simulink model "lab6"  (Simulink 7.7)
settings: Solver=ode45  StartTime=0.0  StopTime=10.0  RelTol=1e-3
settings Model: Creator=Muhammad Ali khan  LastModifiedBy=Muhammad Ali khan

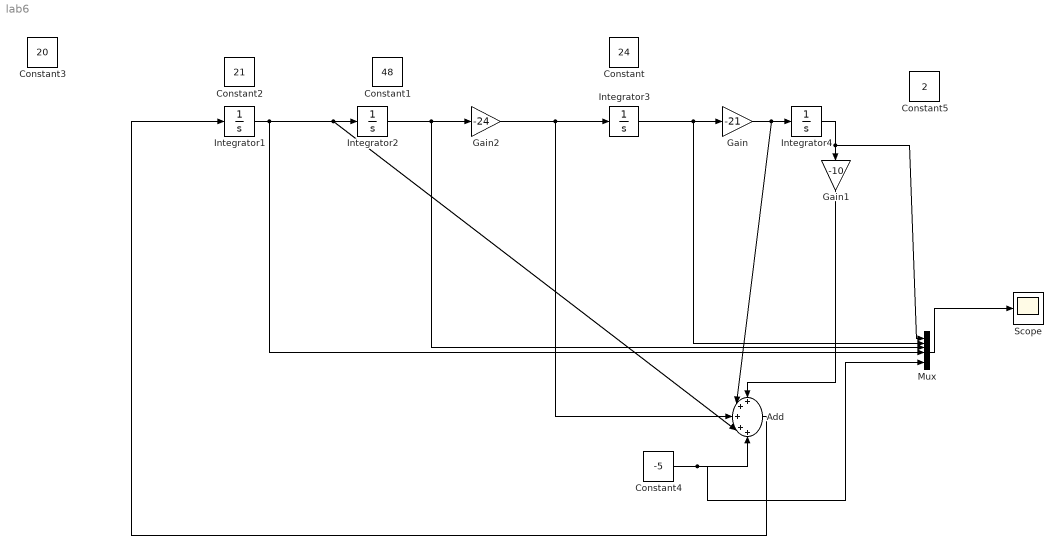
== system lab6 ==
  Add : Sum  Inputs=+++++
  Constant : Constant  Value=24
  Constant1 : Constant  Value=48
  Constant2 : Constant  Value=21
  Constant3 : Constant  Value=20
  Constant4 : Constant  Value=-5
  Constant5 : Constant  Value=2
  Gain : Gain  Gain=-21
  Gain1 : Gain  Gain=-10
  Gain2 : Gain  Gain=-24
  Integrator1 : Integrator  InitialCondition=-2
  Integrator2 : Integrator  InitialCondition=5
  Integrator3 : Integrator  InitialCondition=2
  Integrator4 : Integrator  InitialCondition=1
  Mux : Mux  Inputs=6
  Scope : Scope
  wires:
  Integrator1/1 -> Mux/4, Integrator2/1, Add/4
  Integrator3/1 -> Gain/1, Mux/2
  Integrator4/1 -> Gain1/1, Mux/1
  Integrator2/1 -> Gain2/1, Mux/3
  Gain/1 -> Integrator4/1, Add/2
  Gain2/1 -> Integrator3/1, Add/3
  Constant4/1 -> Mux/6, Add/5
  Mux/1 -> Scope/1
  Gain1/1 -> Add/1
  Add/1 -> Integrator1/1
